simulink model "linear_double_integrator_observer"  (R2025b)
settings: Solver=ode23tb  StartTime=0.0  StopTime=simlength  FixedStep=tc  MaxStep=tc
values from neighbouring files (symbols this model uses):
  kv = Kd(2)/ts_afe    [init_model.m]
  kx = Kd(1)/ts_afe    [init_model.m]
  omega0 = 2*pi*50    (= 314.159265359)    [init_model.m]
  ts_afe = 1/fPWM_AFE/2    (= 0.000125)    [init_model.m]
libraries: linear_double_integrator_observer_ccaller x1
settings Model: SimulationMode=accelerator  Creator=dbagn  LastModifiedBy=dbagn
settings SolverCC: NumberNewtonIterations=3.0  ZeroCrossControl=DisableAll  AlgebraicLoopSolver=TrustRegion  SolverResetMethod=Robust
settings DataIOCC: SaveOutput=off  SignalLogging=off  DSMLogging=off  SaveTime=off  ReturnWorkspaceOutputs=off
settings OptimizationCC: ReuseModelBlockBuffer=off
settings DebuggingCC: UnconnectedInputMsg=warning  UnconnectedOutputMsg=warning  UnconnectedLineMsg=warning
settings ModelReferenceCC: EnableRefExpFcnMdlSchedulingChecks=on
settings SFSimCC: CustomCodeUndefinedFunction=ThrowError  DefaultCustomCodeDeterministicFunctions=All
settings SFSimCC: SimCustomHeaderCode=|
  | #include "rpi.h"
  | #include "mavgflt.h"
  | #include "mavgflt_simulink.h"
  | #include "mavgflts.h"
  | #include "mavgflts_simulink.h"
  | #include "dsmavgflt.h"
  | #include "dsmavgflt_simulink.h"
  | #include "bemf_obsv.h"
  | #include "bemf_obsv_simulink.h"
  | #include "bemf_obsv_load_est.h"
  | #include "bemf_obsv_load_est_simulink.h"
  | #include "dqvector_pi.h"
  | #include "dqvector_pi_simulink.h"
  | #include "sv_pwm_simulink.h"
  | #include "sv_pwm.h"
  | #include "first_harmonic_tracker.h"
  | #include "first_harmonic_tracker_simulink.h"
  | #include "dqpll_thyr.h"
  | #include "dqpll_thyr_simulink.h"
  | #include "dqpll_grid.h"
  | #include "dqpll_grid_simulink.h"
  | #include "linear_double_integrator_observer_simulink.h"
  | #include "linear_double_integrator_observer.h"
settings SFSimCC: SimUserSources=|
  | "rpi.c"
  | "mavgflt_simulink.c"
  | "mavgflt.c"
  | "mavgflts_simulink.c"
  | "mavgflts.c"
  | "dsmavgflt_simulink.c"
  | "dsmavgflt.c"
  | "bemf_obsv_simulink.c"
  | "bemf_obsv.c"
  | "bemf_obsv_load_est_simulink.c"
  | "bemf_obsv_load_est.c"
  | "dqvector_pi.c"
  | "dqvector_pi_simulink.c"
  | "sv_pwm_simulink.c"
  | "sv_pwm.c"
  | "first_harmonic_tracker_simulink.c"
  | "first_harmonic_tracker.c"
  | "dqpll_thyr_simulink.c"
  | "dqpll_thyr.c"
  | "dqpll_grid_simulink.c"
  | "dqpll_grid.c"
  | "linear_double_integrator_observer_simulink.c"
  | "linear_double_integrator_observer.c"
settings SFSimCC: SimUserIncludeDirs=|
  | include
  | src
settings RTWCC: GPUComputeCapability=3.5  DLArmComputeVersion=19.05

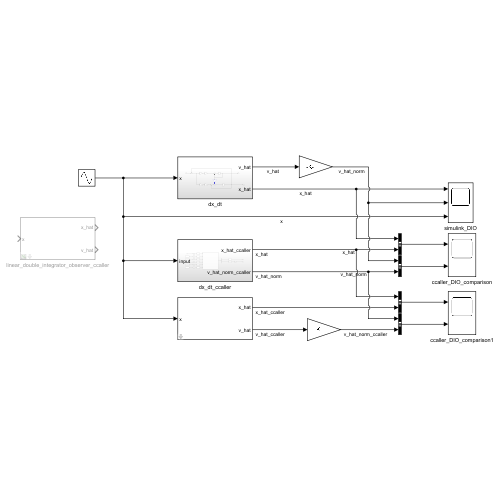
[thumbnail: Simulink's stored preview of the top-level diagram]
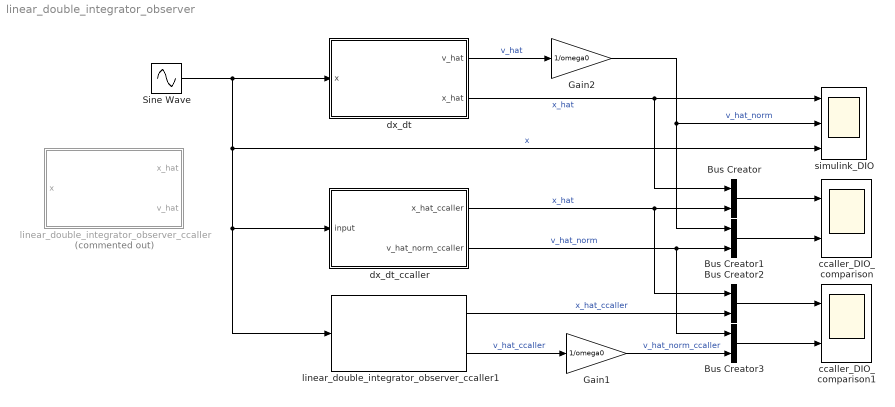
== system linear_double_integrator_observer ==
  Bus Creator{,1..3} (4 alike) : BusCreator  Inputs=2
  Gain1 : Gain  Gain=1/omega0
  Gain2 : Gain  Gain=1/omega0
  Sine Wave : Sin  Frequency=omega0  SampleTime=0
  ccaller_DIO_comparison : Scope  NumInputPorts=2
      settings: ActiveDisplayYMinimum=-1.2688563764095306  ActiveDisplayYMaximum=1.2688563764095306
  ccaller_DIO_comparison1 : Scope  NumInputPorts=2
      settings: ActiveDisplayYMinimum=-1.2688563764095306  ActiveDisplayYMaximum=1.2688563764095306  DataLoggingVariableName=ScopeData2
  dx_dt : Subsystem
  dx_dt_ccaller : Subsystem
  linear_double_integrator_observer_ccaller : Subsystem  Commented=on  mask{kx_m=kx, kv_m=kv, ts_m=ts_afe, time_release=0.05, instance=1, tc_m=ts_afe}
      mask prompts: kx_m "kx"; kv_m "kv"; ts_m "Sampling Time [s]"; time_release "Reset Time Release [s]"; instance "Instance [#]"; tc_m "Sample Time [s] (-1 for inherited)"
  linear_double_integrator_observer_ccaller1 : linear_double_integrator_observer_ccaller/linear_double_integrator_observer_ccaller  kx_m=kx  kv_m=kv  ts_m=ts_afe  time_release=0.05  instance=1  tc_m=ts_afe
  simulink_DIO : Scope  NumInputPorts=3
      settings: ActiveDisplayYMinimum=-1.2826755991631912E+307  ActiveDisplayYMaximum=1.4326922901544779E+306
  wires:
  Sine Wave/1 -> linear_double_integrator_observer_ccaller1/1, dx_dt_ccaller/1(input), simulink_DIO/3, dx_dt/1(x)  "x"
  dx_dt/2(x_hat) -> Bus Creator/1, simulink_DIO/1  "x_hat"
  dx_dt/1(v_hat) -> Gain2/1  "v_hat"
  Gain2/1 -> Bus Creator1/1, simulink_DIO/2  "v_hat_norm"
  Bus Creator/1 -> ccaller_DIO_comparison/1
  Bus Creator1/1 -> ccaller_DIO_comparison/2
  Bus Creator3/1 -> ccaller_DIO_comparison1/2
  Bus Creator2/1 -> ccaller_DIO_comparison1/1
  linear_double_integrator_observer_ccaller1/2 -> Gain1/1  "v_hat_ccaller"
  linear_double_integrator_observer_ccaller1/1 -> Bus Creator2/2  "x_hat_ccaller"
  dx_dt_ccaller/2(v_hat_norm_ccaller) -> Bus Creator3/1, Bus Creator1/2  "v_hat_norm"
  dx_dt_ccaller/1(x_hat_ccaller) -> Bus Creator2/1, Bus Creator/2  "x_hat"
  Gain1/1 -> Bus Creator3/2  "v_hat_norm_ccaller"

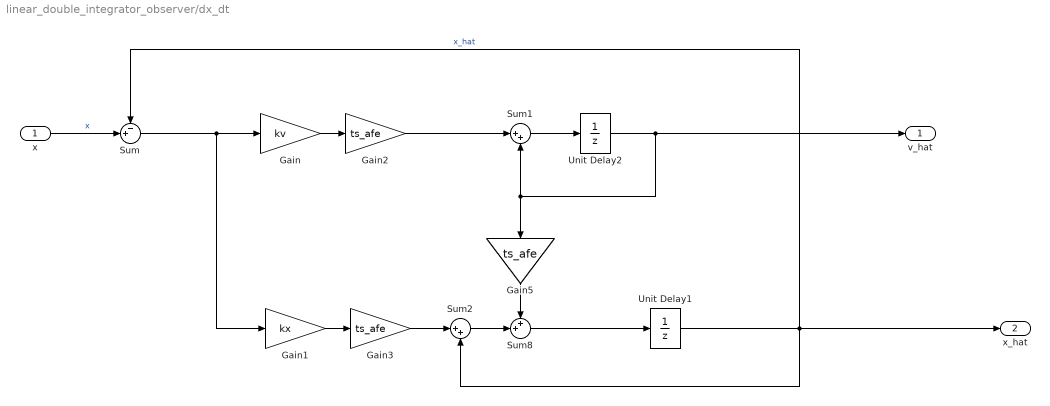
== system linear_double_integrator_observer/dx_dt ==
  x : Inport
  Gain : Gain  Gain=kv
  Gain1 : Gain  Gain=kx
  Gain2 : Gain  Gain=ts_afe
  Gain3 : Gain  Gain=ts_afe
  Gain5 : Gain  Gain=ts_afe
  Sum : Sum  Inputs=-+|
  Sum1 : Sum  Inputs=|++
  Sum2 : Sum  Inputs=|++
  Sum8 : Sum  Inputs=++|
  Unit Delay1 : UnitDelay  SampleTime=ts_afe  HasFrameUpgradeWarning=on
  Unit Delay2 : UnitDelay  SampleTime=ts_afe  HasFrameUpgradeWarning=on
  v_hat : Outport  VectorParamsAs1DForOutWhenUnconnected=off
  x_hat : Outport  Port=2  VectorParamsAs1DForOutWhenUnconnected=off
  wires:
  Gain1/1 -> Gain3/1
  x/1 -> Sum/2  "x"
  Gain5/1 -> Sum8/1
  Sum1/1 -> Unit Delay2/1
  Gain/1 -> Gain2/1
  Sum2/1 -> Sum8/2
  Unit Delay1/1 -> x_hat/1, Sum/1, Sum2/2  "x_hat"
  Sum/1 -> Gain1/1, Gain/1
  Sum8/1 -> Unit Delay1/1
  Unit Delay2/1 -> v_hat/1, Sum1/2, Gain5/1
  Gain2/1 -> Sum1/1
  Gain3/1 -> Sum2/1

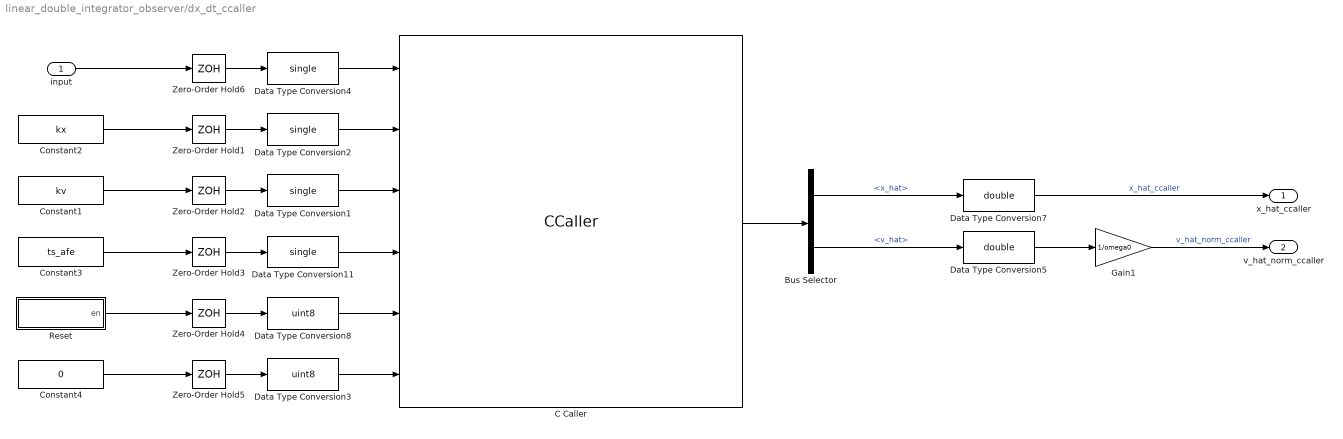
== system linear_double_integrator_observer/dx_dt_ccaller ==
  input : Inport
  Bus Selector : BusSelector  OutputSignals=x_hat,v_hat
  C Caller : CCaller  FunctionName=linear_double_integrator_observer_process_simulink  PortSpecificationStruct="%)30     .    , P   8    (     @         %    \"     <    !     0         %  0 \"0    $    _    07)G3F%M90  4&]R=$YA;64 4V-O<&4     26YD97@     5'EP90      4VEZ90      27-';&]B86P   X    P    !@    @    $          4    (     0    ,    !         !   P!O=70 #@   #     &    \"     0         !0    @    !     P    $         $  # &]U=  .    .     8    (    !          %    \"     $    &     0         0   ...(+3831 chars)"  SampleTime=ts_afe
  Constant1 : Constant  Value=kv
  Constant2 : Constant  Value=kx
  Constant3 : Constant  Value=ts_afe
  Constant4 : Constant  Value=0
  Data Type Conversion{1..2,4,11} (4 alike) : DataTypeConversion  OutDataTypeStr=single  SaturateOnIntegerOverflow=off  RndMeth=Floor
  Data Type Conversion3 : DataTypeConversion  OutDataTypeStr=uint8  SaturateOnIntegerOverflow=off  RndMeth=Floor
  Data Type Conversion5 : DataTypeConversion  OutDataTypeStr=double  SaturateOnIntegerOverflow=off  RndMeth=Floor
  Data Type Conversion7 : DataTypeConversion  OutDataTypeStr=double  SaturateOnIntegerOverflow=off  RndMeth=Floor
  Data Type Conversion8 : DataTypeConversion  OutDataTypeStr=uint8  SaturateOnIntegerOverflow=off  RndMeth=Floor
  Gain1 : Gain  Gain=1/omega0
  Reset : Subsystem
  Zero-Order Hold{1..6} (6 alike) : ZeroOrderHold  SampleTime=ts_afe
  x_hat_ccaller : Outport
  v_hat_norm_ccaller : Outport  Port=2
  wires:
  Zero-Order Hold6/1 -> Data Type Conversion4/1
  input/1 -> Zero-Order Hold6/1
  Constant4/1 -> Zero-Order Hold5/1
  Data Type Conversion8/1 -> C Caller/5
  Zero-Order Hold3/1 -> Data Type Conversion11/1
  Data Type Conversion4/1 -> C Caller/1
  Constant2/1 -> Zero-Order Hold1/1
  Zero-Order Hold2/1 -> Data Type Conversion1/1
  Constant3/1 -> Zero-Order Hold3/1
  Reset/1(en) -> Zero-Order Hold4/1
  Data Type Conversion2/1 -> C Caller/2
  Zero-Order Hold4/1 -> Data Type Conversion8/1
  Data Type Conversion11/1 -> C Caller/4
  Zero-Order Hold1/1 -> Data Type Conversion2/1
  Data Type Conversion3/1 -> C Caller/6
  Constant1/1 -> Zero-Order Hold2/1
  Data Type Conversion1/1 -> C Caller/3
  Zero-Order Hold5/1 -> Data Type Conversion3/1
  Bus Selector/1 -> Data Type Conversion7/1  "<x_hat>"
  C Caller/1 -> Bus Selector/1
  Data Type Conversion7/1 -> x_hat_ccaller/1  "x_hat_ccaller"
  Gain1/1 -> v_hat_norm_ccaller/1  "v_hat_norm_ccaller"
  Data Type Conversion5/1 -> Gain1/1
  Bus Selector/2 -> Data Type Conversion5/1  "<v_hat>"

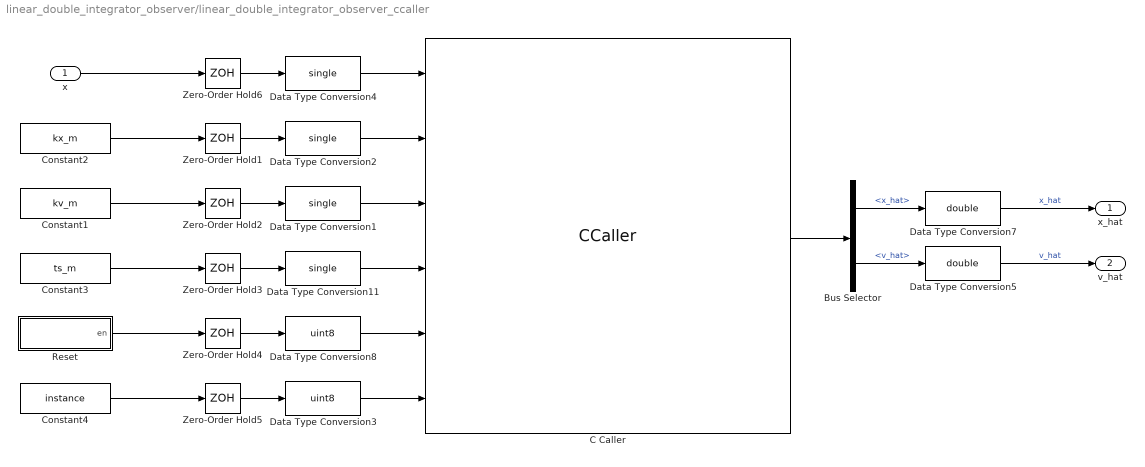
== system linear_double_integrator_observer/linear_double_integrator_observer_ccaller ==
  x : Inport
  Bus Selector : BusSelector  OutputSignals=x_hat,v_hat
  C Caller : CCaller  FunctionName=linear_double_integrator_observer_process_simulink  PortSpecificationStruct="%)30     .    , P   8    (     @         %    \"     <    !     0         %  0 \"0    $    _    07)G3F%M90  4&]R=$YA;64 4V-O<&4     26YD97@     5'EP90      4VEZ90      27-';&]B86P   X    P    !@    @    $          4    (     0    ,    !         !   P!O=70 #@   #     &    \"     0         !0    @    !     P    $         $  # &]U=  .    .     8    (    !          %    \"     $    &     0         0   ...(+3831 chars)"  SampleTime=tc_m
  Constant1 : Constant  Value=kv_m
  Constant2 : Constant  Value=kx_m
  Constant3 : Constant  Value=ts_m
  Constant4 : Constant  Value=instance
  Data Type Conversion{1..2,4,11} (4 alike) : DataTypeConversion  OutDataTypeStr=single  SaturateOnIntegerOverflow=off  RndMeth=Floor
  Data Type Conversion3 : DataTypeConversion  OutDataTypeStr=uint8  SaturateOnIntegerOverflow=off  RndMeth=Floor
  Data Type Conversion5 : DataTypeConversion  OutDataTypeStr=double  SaturateOnIntegerOverflow=off  RndMeth=Floor
  Data Type Conversion7 : DataTypeConversion  OutDataTypeStr=double  SaturateOnIntegerOverflow=off  RndMeth=Floor
  Data Type Conversion8 : DataTypeConversion  OutDataTypeStr=uint8  SaturateOnIntegerOverflow=off  RndMeth=Floor
  Reset : Subsystem
  Zero-Order Hold{1..6} (6 alike) : ZeroOrderHold  SampleTime=tc_m
  x_hat : Outport
  v_hat : Outport  Port=2
  wires:
  Bus Selector/2 -> Data Type Conversion5/1  "<v_hat>"
  Data Type Conversion5/1 -> v_hat/1  "v_hat"
  Data Type Conversion7/1 -> x_hat/1  "x_hat"
  C Caller/1 -> Bus Selector/1
  Bus Selector/1 -> Data Type Conversion7/1  "<x_hat>"
  Zero-Order Hold5/1 -> Data Type Conversion3/1
  Data Type Conversion1/1 -> C Caller/3
  Constant1/1 -> Zero-Order Hold2/1
  Data Type Conversion3/1 -> C Caller/6
  Zero-Order Hold1/1 -> Data Type Conversion2/1
  Data Type Conversion11/1 -> C Caller/4
  Zero-Order Hold4/1 -> Data Type Conversion8/1
  Data Type Conversion2/1 -> C Caller/2
  Reset/1(en) -> Zero-Order Hold4/1
  Constant3/1 -> Zero-Order Hold3/1
  Zero-Order Hold2/1 -> Data Type Conversion1/1
  Constant2/1 -> Zero-Order Hold1/1
  Data Type Conversion4/1 -> C Caller/1
  Zero-Order Hold3/1 -> Data Type Conversion11/1
  Data Type Conversion8/1 -> C Caller/5
  Constant4/1 -> Zero-Order Hold5/1
  x/1 -> Zero-Order Hold6/1
  Zero-Order Hold6/1 -> Data Type Conversion4/1

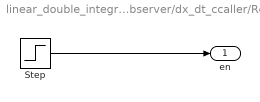
== system linear_double_integrator_observer/dx_dt_ccaller/Reset ==
  Step : Step  Time=0.05  Before=1  After=0  SampleTime=ts_afe
  en : Outport
  wires:
  Step/1 -> en/1

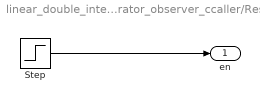
== system linear_double_integrator_observer/linear_double_integrator_observer_ccaller/Reset ==
  Step : Step  Time=time_release  Before=1  After=0
  en : Outport
  wires:
  Step/1 -> en/1
